simulink model "PMSM"  (R2025b)
settings: Solver=VariableStepAuto  StartTime=0.0  StopTime=10.0  RelTol=1e-3
settings Model: Creator=sheik  LastModifiedBy=sheik

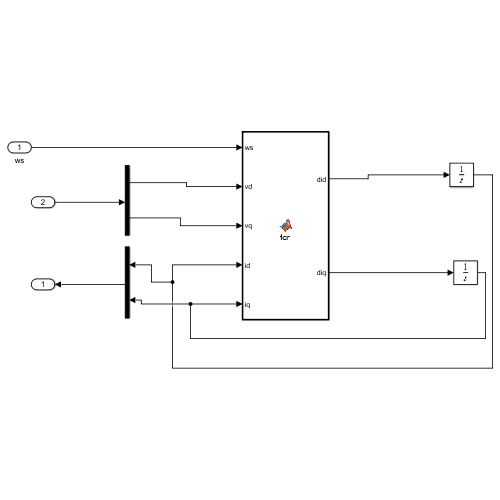
[thumbnail: Simulink's stored preview of the top-level diagram]
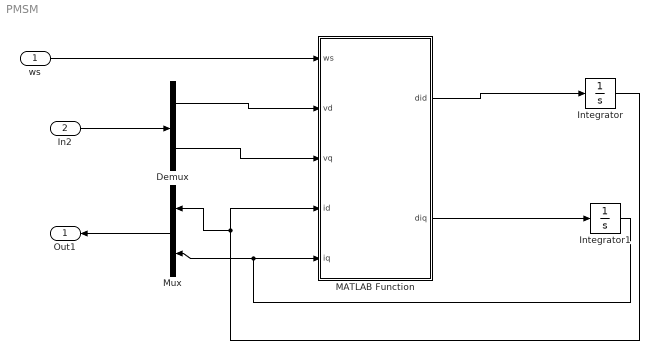
== system PMSM ==
  ws : Inport
  In2 : Inport  Port=2
  Demux : Demux  Outputs=2
  Integrator : Integrator
  Integrator1 : Integrator
  MATLAB Function : MATLAB Function  TreatAsAtomicUnit=on
  Mux : Mux  Inputs=2
  Out1 : Outport
  wires:
  ws/1 -> MATLAB Function/1(ws)
  In2/1 -> Demux/1
  Demux/1 -> MATLAB Function/2(vd)
  Demux/2 -> MATLAB Function/3(vq)
  MATLAB Function/1(did) -> Integrator/1
  MATLAB Function/2(diq) -> Integrator1/1
  Integrator/1 -> MATLAB Function/4(id), Mux/1
  Integrator1/1 -> MATLAB Function/5(iq), Mux/2
  Mux/1 -> Out1/1

== matlab function PMSM/MATLAB Function ==
  data: ws input; did output; vd input; vq input; id input; iq input; diq output
function [did,diq] = fcn(ws,vd,vq,id,iq)
Ld=1e-4;
Lq=1e-3;
Rs=0.00475;
phi=0.23;
did=ws*(Lq/Ld)*iq-(Rs/Ld)*id+(1/Ld)*vd;
diq=-ws*(1/Lq)*phi-ws*(Ld/Lq)*id-(Rs/Lq)*iq+(1/Lq)*vq;
